simulink model "MPC"  (R2024b)
settings: Solver=ode4  StartTime=0.0  StopTime=tsim  FixedStep=baseRate  RelTol=1e-6  AbsTol=1e-6
values from neighbouring files (symbols this model uses):
  C = [cos(theta), -sin(theta) ... (first row only)    [Run_Initializer.m]    (also in plotBatch.m = quat2Rotm(q','scalarFirst'))
  camera_FOV = 40*d2r    (= 0.698131700798)    [Run_Initializer.m]
  camera_offset = [0.145, 0.087]'    [Run_Initializer.m]
  docking_face = [0 1]'    [Run_Initializer.m]
  docking_offset = [0 0 0]'    [Run_Initializer.m]
  eta = 0.7    [Run_Initializer.m]
  F_t = [kron(eye(N_h),  [zeros(2,3), eye(2), zeros(2,4)]) ... (first row only)    [Run_Initializer.m]
  f_t = [kron(ones(N_h, 1), [xLength yLength]' - edge_buffer) ... (first row only)    [Run_Initializer.m]
  F_u = [kron(eye(N_h),  [eye(3), zeros(3,6)]) ... (first row only)    [Run_Initializer.m]
  f_u = kron(ones(2*N_h, 1), u_max')    [Run_Initializer.m]
  F_v = [kron(eye(N_h),  [zeros(1,5), 1, zeros(1,3)]) ... (first row only)    [Run_Initializer.m]
  gamma = 0.95    [Run_Initializer.m]
  Gamma1_el = 0.12    [Run_Initializer.m]
  Gamma1_sh = 0.005    [Run_Initializer.m]
  Gamma1_wr = 0.025    [Run_Initializer.m]
  Gamma2_el = 5    [Run_Initializer.m]
  Gamma2_sh = 5    [Run_Initializer.m]
  Gamma2_wr = 5    [Run_Initializer.m]
  Gamma3_el = 10    [Run_Initializer.m]
  Gamma3_sh = 40    [Run_Initializer.m]
  Gamma3_wr = 40    [Run_Initializer.m]
  Gamma4_el = 0.039    [Run_Initializer.m]
  Gamma4_sh = 0.015    [Run_Initializer.m]
  Gamma4_wr = 0.029    [Run_Initializer.m]
  Gamma5_el = 800    [Run_Initializer.m]
  Gamma5_sh = 800    [Run_Initializer.m]
  Gamma5_wr = 800    [Run_Initializer.m]
  Gamma6_el = 0.000001    (= 1e-06)    [Run_Initializer.m]
  Gamma6_sh = 0.005    [Run_Initializer.m]
  Gamma6_wr = 0.02    [Run_Initializer.m]
  H = kron(eye(N_h), [R, zeros(3,6); zeros(6,3), Q])    [Run_Initializer.m]
  IBLACK = 0.1996    [unpackData.m]
  IRED = 0.1982    [unpackData.m]
  J = sum(wp*posErr + wt*angErr)    [find_transformation.m]
  Kd_elarm = 0.8    [Run_Initializer.m]
  Kd_sharm = 1.0    (= 1)    [Run_Initializer.m]
  Kd_wrarm = 0.6    [Run_Initializer.m]
  Kp_elarm = 1.2    [Run_Initializer.m]
  Kp_sharm = 1.5    [Run_Initializer.m]
  Kp_wrarm = 1.0    (= 1)    [Run_Initializer.m]
  m = m + 5    (= 4)    [unpackData.m]
  M = diag([1/m; 1/m; 1/I])    [unpackData.m]
  maxd = [d1 ... (first row only)    [Run_Initializer.m]
  mBLACK = 11.3620    (= 11.362)    [unpackData.m]
  mRED = 11.2970    (= 11.297)    [unpackData.m]
  N = size(rel,1)    [plotBatch.m]    (also in unpackData.m = 0)
  p = [0 obj.pos(k,:)]    [SparseState6DOF.m]
  PDQ = blkdiag(20*eye(3),eye(3), 20*eye(3),eye(3))    [Run_Initializer.m]
  PQ = blkdiag(20*eye(6),eye(6))    [Run_Initializer.m]
  PR = blkdiag(20*eye(3), eye(6), 0.0001*eye(3))    [Run_Initializer.m]
  PWMFreq = 5    [Run_Initializer.m]
  Q = diag([100 100 100 300 300 300])    [Run_Initializer.m]    (also in unpackData.m = blkdiag(0.0001*eye(2), 0.00001))
  R = diag([200 200 200])    [Run_Initializer.m]    (also in plotBatch.m = C3(yaw); unpackData.m = diag([6;6;6]))
  r_hold_obs = 1.1*sqrt(2)*0.3.*[1 1]    [Run_Initializer.m]
  r_hold_tar_min = [0.8; (0.3+0.05)]    [Run_Initializer.m]
  rho = 0.98    [Run_Initializer.m]
  T_d = 2    [Run_Initializer.m]
  T_max = 0.15    [Run_Initializer.m]
  Tz_lim_elarm = .1    (= 0.1)    [Run_Initializer.m]
  Tz_lim_sharm = .1    (= 0.1)    [Run_Initializer.m]
  Tz_lim_wrarm = .1    (= 0.1)    [Run_Initializer.m]
  use_LOS_constr = 1    [Run_Initializer.m]
  use_table_constr = 1    [Run_Initializer.m]
  x_BLACK_0 = [(1/3)*xLength (1/3)*yLength-0.2 280*d2r 0.01 0.005 1.88*d2r]'    [Run_Initializer.m]
  x_BLUE_0 = [0 0 0 0 0 0]'    [Run_Initializer.m]
  zeta = 10*d2r    (= 0.174532925199)    [Run_Initializer.m]
undefined symbols (not defined in the file or in its folder): a1, a2, a3, alpha, alpha_m, alpha_t, alphas, alphas_t, alphat, Am, b, b0, b1, b2, b3, baseRate, Bm, c, c1, c1t, c2, c2t, Cm, d, dataRate, DiscIntNeverNeededParam, Dm, drop_states_ARM, drop_states_BLACK, drop_states_BLUE, drop_states_RED, epsilon, epsilont, F_black_X_nominal, F_black_Y_nominal, F_blue_X_nominal, F_blue_Y_nominal, F_max, F_red_X_nominal, F_red_Y_nominal, F_thrusters_BLACK, F_thrusters_BLUE, F_thrusters_RED, gamma_I, gamma_I_t, gamma_P, gamma_P_t, home_states_BLACK, home_states_BLUE, home_states_RED, IBLUE, IDIST, IEE, init_states_BLACK, init_states_BLUE, init_states_RED, IPROX, k, K, k1 ... (+62)
libraries: simulink x33, nvidiaSharedBlocks x13, slpidlib x6, MainLibrary x5, dspsigops x3, dspinverses x3, nvidiaIMUSensorslib x1
(part 11 of 12)

== matlab function MPC/4 - Control/Default PD Control (RED)/Sat/MATLAB Function5 ==
  data: q2 input; u input; saturation output; e parameter; T_max parameter; d parameter; J parameter
function saturation = fcn(q2,u,e, T_max, d, J)

if u >= e
    u = e;
elseif u <= -1*e
    u = -1*e;
else
    u = u;
end

u = d*q2*J + u;

if u >= T_max
    u = T_max;
elseif u <= -1*T_max
    u = -1*T_max;
else
    u = u;
end

saturation = u;

== matlab function MPC/4 - Control/Default PD Control (RED)/USC/MATLAB Function ==
  data: q1 input; k_dot output; q2 input; c1 parameter; c2 parameter
function k_dot = fcn(q1,q2,c1, c2)
k_dot = (q1*c1 + q2*c2)^2;
end

== matlab function MPC/4 - Control/Default PD Control (RED)/USC/MATLAB Function1 ==
  data: k input; q2 input; q1 input; u output; c1 parameter; c2 parameter
function u = fcn(k,q2,q1,c1, c2)
u = log(k)*(q1*c1 + q2*c2)*cos(sqrt(log(k)));
end

== matlab function MPC/4 - Control/Default PD Control (RED)/USC/MATLAB Function2 ==
  data: q1 input; k_dot output; q2 input; c1 parameter; c2 parameter
function k_dot = fcn(q1,q2,c1, c2)
k_dot = (q1*c1 + q2*c2)^2;
end

== matlab function MPC/4 - Control/Default PD Control (RED)/USC/MATLAB Function3 ==
  data: k input; q2 input; q1 input; u output; c1 parameter; c2 parameter
function u = fcn(k,q2,q1,c1, c2)
u = log(k)*(q1*c1 + q2*c2)*cos(sqrt(log(k)));
end

== matlab function MPC/4 - Control/Default PD Control (RED)/USC/MATLAB Function4 ==
  data: q1 input; k_dot output; q2 input; c1t parameter; c2t parameter
function k_dot = fcn(q1,q2,c1t, c2t)
k_dot = (q1*c1t + q2*c2t)^2;
end

== matlab function MPC/4 - Control/Default PD Control (RED)/USC/MATLAB Function5 ==
  data: k input; q2 input; q1 input; u output; c1t parameter; c2t parameter
function u = fcn(k,q2,q1,c1t, c2t)
u = log(k)*(q1*c1t + q2*c2t)*cos(sqrt(log(k)));
end

== matlab function MPC/4 - Control/Default PD Control (RED)/SAC/SAC_CTL/Position/Storage/MATLAB Function4 ==
  data: u input; y1 output; y2 output
function [y1,y2] = fcn(u)

y1 = u(1,:);
y2 = u(2,:);
end

== matlab function MPC/3 - Navigation/Subsystem/Filter Error/MATLAB Function2 ==
  data: true input; y output; est input
function y = fcn(true, est)
true(1:4) = normalizeQuat(true(1:4),'scalarFirst');
q = quatInv(true(1:4),'scalarFirst');
q = quatMultiply(q,est(1:4),'scalarFirst');
q = smallQuat(q,'scalarFirst');
mrp = quat2mrp(q,1,1,'scalarFirst');

temp = true(5:end) - est(5:end);

y = [mrp(3); temp(1:2); temp(6); temp(7:8)];

== matlab function MPC/3 - Navigation/Subsystem/Filter Error/MATLAB Function3 ==
  data: u input; y output; data input
function y = fcn(u, data)
y = quatMultiply(data,u,'scalarFirst');
y = smallQuat(y,'scalarFirst');

== matlab function MPC/3 - Navigation/Subsystem/Filter Error/MATLAB Function4 ==
  data: true input; y output; est input
function y = fcn(true, est)
true(1:4) = normalizeQuat(true(1:4),'scalarFirst');
q = quatInv(true(1:4),'scalarFirst');
q = quatMultiply(q,est(1:4),'scalarFirst');
q = smallQuat(q,'scalarFirst');
mrp = quat2mrp(q,1,1,'scalarFirst');

temp = true(5:end) - est(5:end);

y = [mrp(3); temp(1:2); temp(6); temp(7:8)];

== matlab function MPC/3 - Navigation/Subsystem/Filter Error/MATLAB Function5 ==
  data: q input; y output; v input; x input
function y = fcn(q, v, x)
t = 0.75;
t = 0;
a = [0;0;1;t*pi/180];
d = axang2Quat(a,'scalarFirst');
d = normalizeQuat(d,'scalarFirst');
q = normalizeQuat(q,'scalarFirst');
q = quatMultiply(d,q,'scalarFirst');
v = quatRotate(q,v,'scalarFirst');
y = v + x;

== matlab function MPC/3 - Navigation/Subsystem/Filter Error/MATLAB Function6 ==
  data: true input; y output; est input
function y = fcn(true, est)
true(1:4) = normalizeQuat(true(1:4),'scalarFirst');
q = quatInv(true(1:4),'scalarFirst');
q = quatMultiply(q,est(1:4),'scalarFirst');
q = smallQuat(q,'scalarFirst');
mrp = quat2mrp(q,1,1,'scalarFirst');

temp = true(5:end) - est(5:end);

y = [mrp(3); temp(1:2); temp(6); temp(7:8)];

== matlab function MPC/3 - Navigation/Subsystem/Filter Error/MATLAB Function7 ==
  data: true input; y output; est input
function y = fcn(true, est)
true(1:4) = normalizeQuat(true(1:4),'scalarFirst');
q = quatInv(true(1:4),'scalarFirst');
q = quatMultiply(q,est(1:4),'scalarFirst');
q = smallQuat(q,'scalarFirst');
mrp = quat2mrp(q,1,1,'scalarFirst');

temp = true(5:end) - est(5:end);
y = [mrp(3); temp(1); temp(2);];

== matlab function MPC/3 - Navigation/Subsystem/Filter Error/MATLAB Function8 ==
  data: true input; y output; est input
function y = fcn(true, est)
true(1:4) = normalizeQuat(true(1:4),'scalarFirst');
q = quatInv(true(1:4),'scalarFirst');
q = quatMultiply(q,est(1:4),'scalarFirst');
q = smallQuat(q,'scalarFirst');
mrp = quat2mrp(q,1,1,'scalarFirst');

temp = true(5:end) - est(5:end);

y = [mrp(3); temp(1:2); temp(6); temp(7:8)];

== matlab function MPC/3 - Navigation/Subsystem/Representations/MATLAB Function ==
  data: u input; dq output; q output; R output; x output; v output; w output; yaw output
function [dq,q,R,x,v,w,yaw] = fcn(u)
    v = u(7:9);
    w = u(10:12);
    x = u(1:3);
    R = C3(u(6));
    yaw = u(6);
    T = [R, x; zeros(1,3), 1];
    T = htformInverse(T);
    q = rotm2Quat(R,'scalarFirst');
    q = smallQuat(q,'scalarFirst');
    dq = htform2Dq(T,'scalarFirst');
end

== matlab function MPC/3 - Navigation/Subsystem/Representations1/MATLAB Function ==
  data: u input; dq output; q output; R output; x output; v output; w output; yaw output
function [dq,q,R,x,v,w,yaw] = fcn(u)
    v = u(7:9);
    w = u(10:12);
    x = u(1:3);
    R = C3(u(6));
    yaw = u(6);
    T = [R, x; zeros(1,3), 1];
    q = rotm2Quat(R,'scalarFirst');
    q = smallQuat(q,'scalarFirst');
    dq = htform2Dq(T,'scalarFirst');
end

== matlab function MPC/2 - Guidance/Default APF PPL (RED)/MATLAB Function ==
  data: desiredPosition input; currentPosition output; currentPosition input; obstacles input; attractiveGain input; repulsiveGain input; influenceRange input; angularGain input; baseRate parameter
function currentPosition = APFPathPlanner(desiredPosition, currentPosition, obstacles, attractiveGain, repulsiveGain, influenceRange, angularGain, baseRate)
    % APFPathPlanner for real-time path planning in Simulink
    % Controls X, Y, and Attitude (Theta)
    % currentPosition: [x, y, theta]
    % desiredPosition: [x, y, theta]
    % obstacles: Nx2 matrix of obstacle positions [x, y]
    % attractiveGain: Scalar for attractive force
    % repulsiveGain: Scalar for repulsive force
    % influenceRange: Scalar, range for obstacle influence
    % angularGain: Scalar for angular adjustment


    % Position control for X and Y
    attractiveForce = attractiveGain * (desiredPosition(1:2) - currentPosition(1:2));
    repulsiveForce = zeros(1, 2);

    % % Repulsive force from obstacles
    for i = 1:size(obstacles, 1)
        obstaclePos = obstacles(i, :);
        distanceToObstacle = norm(currentPosition(1:2) - obstaclePos);

        if distanceToObstacle < influenceRange
            directionFromObstacle = (currentPosition(1:2) - obstaclePos) / distanceToObstacle;
            magnitude = repulsiveGain * (1 / distanceToObstacle - 1 / influenceRange) * (1 / distanceToObstacle^2);
            repulsiveForce = repulsiveForce + magnitude * directionFromObstacle;
        end
    end

    % Combine attractive and repulsive forces
    totalForce = attractiveForce + repulsiveForce;

    % Update X and Y position
    deltaT = baseRate;
    newPosition = currentPosition(1:2) + deltaT * totalForce;

    % Attitude control for Theta
    angularDifference = atan2(sin(desiredPosition(3) - currentPosition(3)), cos(desiredPosition(3) - currentPosition(3)));
    newTheta = currentPosition(3) + angularGain * angularDifference * deltaT;

    % Normalize newTheta to be within -pi to pi
    newTheta = atan2(sin(newTheta), cos(newTheta));

    % Update currentPosition with new position and attitude
    currentPosition = [newPosition, newTheta];

end

== matlab function MPC/3 - Navigation/Subsystem/MATLAB Function ==
  data: u input; states output
function states = fcn(u)

x = u(1);
y = u(2);
z = 0;
roll = 0;
pitch = 0;
yaw = u(3);
dx = u(4);
dy = u(5);
dz = 0;
droll = 0;
dpitch = 0;
dyaw = u(6);

states = [x; y; z; ...
          roll; pitch; yaw; ...
          dx; dy; dz; ...
          droll; dpitch; dyaw];

== matlab function MPC/3 - Navigation/Subsystem/MATLAB Function1 ==
  data: u input; states output
function states = fcn(u)

x = u(1);
y = u(2);
z = 0;
roll = 0;
pitch = 0;
yaw = u(3);
dx = u(4);
dy = u(5);
dz = 0;
droll = 0;
dpitch = 0;
dyaw = u(6);

states = [x; y; z; ...
          roll; pitch; yaw; ...
          dx; dy; dz; ...
          droll; dpitch; dyaw];

== matlab function MPC/PhaseSpace Camera Code/Use Hardware to Obtain States/Store RED Data/Subsystem1/Enabled Subsystem/MATLAB Function ==
  data: y input; dy output; dt input; tau input; dy_prev input; ema_prev input; ema output
function [dy, ema] = realtime_derivative_ema(y, dt, tau, dy_prev, ema_prev)
    % Inputs:
    % y: Current measurement
    % dt: Time step
    % alpha: Smoothing factor (e.g., 0.1)

    alpha = 1 - exp(-dt / tau);
        
    % Update EMA
    ema = alpha.*y + (1 - alpha).*ema_prev;
    
    % Compute derivative
    dy = (ema - ema_prev)./dt;
    
end

== matlab function MPC/Simulate Plant Dynamics/BLACK Dynamics/Calculated & Store Measured States/Subsystem2/Enabled Subsystem/MATLAB Function ==
  data: y input; dy output; dt input; tau input; dy_prev input; ema_prev input; ema output
function [dy, ema] = realtime_derivative_ema(y, dt, tau, dy_prev, ema_prev)
    % Inputs:
    % y: Current measurement
    % dt: Time step
    % alpha: Smoothing factor (e.g., 0.1)

    alpha = 1 - exp(-dt / tau);
        
    % Update EMA
    ema = alpha.*y + (1 - alpha).*ema_prev;
    
    % Compute derivative
    dy = (ema - ema_prev)./dt;
    
end

== matlab function MPC/Simulate Plant Dynamics/RED and ARM Dynamics/RED + ARM/Coriolis Function1 ==
  data: a1 parameter; a2 parameter; a3 parameter; b0 parameter; b1 parameter; b2 parameter; mPROX parameter; mDIST parameter; mEE parameter; Phi parameter; CoriolisS output; x input
function CoriolisS = CoriolisFunc3LINK(a1,a2,a3,b0,b1,b2,mPROX,mDIST,mEE,Phi,x)
%CORIOLISFUNC3LINK
%    CORIOLISS = CORIOLISFUNC3LINK(A1,A2,A3,B0,B1,B2,mPROX,mDIST,mEE,PHI,Q0,Q1,Q2,Q3,Q0_DOT,Q1_DOT,Q2_DOT,Q3_DOT)

%    This function was generated by the Symbolic Math Toolbox version 8.0.
%    05-Nov-2017 11:48:44

q0 = x(3);
q1 = x(4);
q2 = x(5);
q3 = x(6);

q0_dot = x(9);
q1_dot = x(10);
q2_dot = x(11);
q3_dot = x(12);

t2 = a1+b1;
t3 = a1.*mPROX;
t4 = mDIST.*t2;
t5 = mEE.*t2;
t6 = t3+t4+t5;
t7 = a2.*mDIST;
t8 = a2+b2;
t9 = mEE.*t8;
t10 = t7+t9;
t11 = pi.*(1.0./2.0);
t12 = q0_dot.*t6;
t13 = q1_dot.*t6;
t14 = q0+q1+t11;
t15 = cos(t14);
t16 = t12+t13;
t17 = q0_dot.*t10;
t18 = q1_dot.*t10;
t19 = q2_dot.*t10;
t20 = q0+q1+q2+t11;
t21 = cos(t20);
t22 = t17+t18+t19;
t23 = a3.*mEE.*q0_dot;
t24 = a3.*mEE.*q1_dot;
t25 = a3.*mEE.*q2_dot;
t26 = a3.*mEE.*q3_dot;
t27 = q0+q1+q2+q3+t11;
t28 = cos(t27);
t29 = t23+t24+t25+t26;
t30 = b0.*mPROX;
t31 = b0.*mDIST;
t32 = b0.*mEE;
t33 = t30+t31+t32;
t34 = (pi/2-Phi)+q0;
t35 = sin(t14);
t36 = sin(t20);
t37 = sin(t27);
t38 = q0_dot+q1_dot+q2_dot+q3_dot;
t39 = q0+q1+q2+q3;
t40 = a1.*b0.*mPROX.*q1_dot;
t41 = a1.*b0.*mDIST.*q1_dot;
t42 = a1.*b0.*mEE.*q1_dot;
t43 = b0.*b1.*mDIST.*q1_dot;
t44 = b0.*b1.*mEE.*q1_dot;
t45 = (pi/2-Phi)-q1;
t46 = cos(t45);
t47 = a2.*b0.*mDIST.*q1_dot;
t48 = a2.*b0.*mDIST.*q2_dot;
t49 = a2.*b0.*mEE.*q1_dot;
t50 = a2.*b0.*mEE.*q2_dot;
t51 = b0.*b2.*mEE.*q1_dot;
t52 = b0.*b2.*mEE.*q2_dot;
t53 = -(pi/2-Phi)+q1+q2;
t54 = cos(t53);
t55 = a3.*b0.*mEE.*q1_dot;
t56 = a3.*b0.*mEE.*q2_dot;
t57 = a3.*b0.*mEE.*q3_dot;
t58 = -(pi/2-Phi)+q1+q2+q3;
t59 = cos(t58);
t60 = a2.*b1.*mDIST.*q2_dot;
t61 = a1.*b2.*mEE.*q2_dot;
t62 = a2.*b1.*mEE.*q2_dot;
t63 = b1.*b2.*mEE.*q2_dot;
t64 = a1.*a2.*mDIST.*q2_dot;
t65 = a1.*a2.*mEE.*q2_dot;
t66 = sin(q2);
t67 = t60+t61+t62+t63+t64+t65;
t68 = a3.*b2.*mEE.*q3_dot;
t69 = a2.*a3.*mEE.*q3_dot;
t70 = sin(q3);
t71 = t68+t69;
t72 = a3.*b1.*mEE.*q2_dot;
t73 = a3.*b1.*mEE.*q3_dot;
t74 = a1.*a3.*mEE.*q2_dot;
t75 = a1.*a3.*mEE.*q3_dot;
t76 = q2+q3;
t77 = sin(t76);
t78 = t72+t73+t74+t75;
t79 = a2.*b0.*mDIST.*q0_dot;
t80 = a2.*b0.*mEE.*q0_dot;
t81 = b0.*b2.*mEE.*q0_dot;
t82 = t47+t48+t49+t50+t51+t52+t79+t80+t81;
t83 = a3.*b0.*mEE.*q0_dot;
t84 = t55+t56+t57+t83;
t85 = a1.*b0.*mPROX.*q0_dot;
t86 = a1.*b0.*mDIST.*q0_dot;
t87 = a1.*b0.*mEE.*q0_dot;
t88 = b0.*b1.*mDIST.*q0_dot;
t89 = b0.*b1.*mEE.*q0_dot;
t90 = a2.*b1.*mDIST.*q0_dot;
t91 = a1.*b2.*mEE.*q0_dot;
t92 = a2.*b1.*mDIST.*q1_dot;
t93 = a2.*b1.*mEE.*q0_dot;
t94 = a1.*b2.*mEE.*q1_dot;
t95 = a2.*b1.*mEE.*q1_dot;
t96 = b1.*b2.*mEE.*q0_dot;
t97 = b1.*b2.*mEE.*q1_dot;
t98 = a1.*a2.*mDIST.*q0_dot;
t99 = a1.*a2.*mDIST.*q1_dot;
t100 = a1.*a2.*mEE.*q0_dot;
t101 = a1.*a2.*mEE.*q1_dot;
t102 = t60+t61+t62+t63+t64+t65+t90+t91+t92+t93+t94+t95+t96+t97+t98+t99+t100+t101;
t103 = a3.*b1.*mEE.*q0_dot;
t104 = a3.*b1.*mEE.*q1_dot;
t105 = a1.*a3.*mEE.*q0_dot;
t106 = a1.*a3.*mEE.*q1_dot;
t107 = t72+t73+t74+t75+t103+t104+t105+t106;
t108 = t79+t80+t81;
t109 = t54.*t108;
t110 = t59.*t83;
t111 = t90+t91+t92+t93+t94+t95+t96+t97+t98+t99+t100+t101;
t112 = t66.*t111;
t113 = t103+t104+t105+t106;
t114 = t77.*t113;
t115 = a2.*q0_dot;
t116 = a2.*q1_dot;
t117 = a2.*q2_dot;
t118 = b2.*q0_dot;
t119 = b2.*q1_dot;
t120 = b2.*q2_dot;
t121 = t115+t116+t117+t118+t119+t120;
t122 = a3.*mEE.*t70.*t121;
t123 = a1.*q0_dot;
t124 = a1.*q1_dot;
t125 = b1.*q0_dot;
t126 = b1.*q1_dot;
t127 = t123+t124+t125+t126;
t128 = a3.*mEE.*t77.*t127;
CoriolisS = reshape([0.0,0.0,0.0,0.0,0.0,0.0,0.0,0.0,0.0,0.0,0.0,0.0,-t15.*t16-t21.*t22-t28.*t29-q0_dot.*t33.*cos(t34),-t16.*t35-t22.*t36-t29.*t37-q0_dot.*t33.*sin(t34),-t66.*t67-t70.*t71-t77.*t78-t46.*(t40+t41+t42+t43+t44)-t59.*(t55+t56+t57)-t54.*(t47+t48+t49+t50+t51+t52),t109+t110-t66.*t67-t70.*t71-t77.*t78+t46.*(t85+t86+t87+t88+t89),t109+t110+t112+t114-t70.*t71,t110+t122+t128,-t15.*t16-t21.*t22-t28.*t29,-t16.*t35-t22.*t36-t29.*t37,-t66.*t67-t54.*t82-t70.*t71-t59.*t84-t77.*t78-t46.*(t40+t41+t42+t43+t44+t85+t86+t87+t88+t89),-t66.*t67-t70.*t71-t77.*t78,t112+t114-t70.*t71,t122+t128,-t21.*t22-t28.*t29,-t22.*t36-t29.*t37,-t54.*t82-t70.*t71-t59.*t84-t66.*t102-t77.*t107,-t70.*t71-t66.*t102-t77.*t107,-a3.*mEE.*q3_dot.*t8.*t70,a3.*mEE.*t8.*t70.*(q0_dot+q1_dot+q2_dot),a3.*mEE.*t38.*sin(t39),-a3.*mEE.*t38.*cos(t39),-a3.*b0.*mEE.*t38.*t59-a3.*mEE.*t8.*t38.*t70-a3.*mEE.*t2.*t38.*t77,-a3.*mEE.*t8.*t38.*t70-a3.*mEE.*t2.*t38.*t77,-a3.*mEE.*t8.*t38.*t70,0.0],[6,6]);
end

== matlab function MPC/Simulate Plant Dynamics/BLACK Dynamics/Data @ Measurement Rate/Calculate True Time Step/MATLAB Function ==
  data: dt input; dt_out output; dataRate input
function dt_out = CheckforInvalidTime(dt, dataRate)

    if dt <= 0

        dt_out = dataRate;

    else

        dt_out = dt;

    end


end

== matlab function MPC/Simulate Plant Dynamics/RED and ARM Dynamics/RED + ARM/Inertia Function 1 ==
  data: mRED parameter; IRED parameter; Phi parameter; b0 parameter; a1 parameter; b1 parameter; a2 parameter; b2 parameter; a3 parameter; b3 parameter; mPROX parameter; mDIST parameter; mEE parameter; IPROX parameter; IDIST parameter; InertiaS output; x input; IEE parameter
function InertiaS = InertiaFunc3LINK(mRED, IRED, Phi, b0, a1, b1, a2, b2, a3, b3, mPROX, mDIST, mEE, IPROX, IDIST, x, IEE)

    q0 = x(3);
    q1 = x(4);
    q2 = x(5);
    q3 = x(6);
    
    t2 = a1+b1;
    t3 = a1.*mPROX;
    t4 = mDIST.*t2;
    t5 = mEE.*t2;
    t6 = q0+q1;
    t7 = cos(t6);
    t8 = t3+t4+t5;
    t9 = a2.*mDIST;
    t10 = a2+b2;
    t11 = mEE.*t10;
    t12 = q0+q1+q2;
    t13 = cos(t12);
    t14 = t9+t11;
    t15 = q0+q1+q2+q3;
    t16 = cos(t15);
    t17 = mRED+mPROX+mDIST+mEE;
    t18 = b0.*mPROX;
    t19 = b0.*mDIST;
    t20 = b0.*mEE;
    t21 = t18+t19+t20;
    t22 = (pi/2-Phi)+q0;
    t23 = sin(t6);
    t24 = sin(t12);
    t25 = sin(t15);
    t26 = a2.*mEE;
    t27 = b2.*mEE;
    t28 = t9+t26+t27;
    t29 = sin(t22);
    t86 = t7.*t8;
    t87 = t13.*t14;
    t88 = a3.*mEE.*t16;
    t30 = -t86-t87-t88-t21.*t29;
    t31 = cos(t22);
    t32 = t21.*t31;
    t89 = t8.*t23;
    t90 = t14.*t24;
    t91 = a3.*mEE.*t25;
    t33 = t32-t89-t90-t91;
    t34 = a1.^2;
    t35 = a2.^2;
    t36 = b0.^2;
    t37 = b1.^2;
    t38 = a1.*a2.*mDIST.*2.0;
    t39 = a1.*a2.*mEE.*2.0;
    t40 = a2.*b1.*mDIST.*2.0;
    t41 = a1.*b2.*mEE.*2.0;
    t42 = a2.*b1.*mEE.*2.0;
    t43 = b1.*b2.*mEE.*2.0;
    t44 = t38+t39+t40+t41+t42+t43;
    t45 = cos(q2);
    t46 = t44.*t45;
    t47 = a2.*a3.*mEE.*2.0;
    t48 = a3.*b2.*mEE.*2.0;
    t49 = t47+t48;
    t50 = cos(q3);
    t51 = t49.*t50;
    t52 = a1.*a3.*mEE.*2.0;
    t53 = a3.*b1.*mEE.*2.0;
    t54 = t52+t53;
    t55 = q2+q3;
    t56 = cos(t55);
    t57 = t54.*t56;
    t58 = (pi/2-Phi)-q1;
    t59 = sin(t58);
    t60 = -(pi/2-Phi)+q1+q2;
    t61 = sin(t60);
    t62 = -(pi/2-Phi)+q1+q2+q3;
    t63 = sin(t62);
    t64 = mPROX.*t34;
    t65 = mDIST.*t34;
    t66 = mEE.*t34;
    t67 = mDIST.*t35;
    t68 = mEE.*t35;
    t69 = a3.^2;
    t70 = mEE.*t69;
    t71 = mDIST.*t37;
    t72 = mEE.*t37;
    t73 = b2.^2;
    t74 = mEE.*t73;
    t75 = a1.*b1.*mDIST.*2.0;
    t76 = a1.*b1.*mEE.*2.0;
    t77 = a2.*b2.*mEE.*2.0;
    t78 = a2.*b0.*mDIST;
    t79 = a2.*b0.*mEE;
    t80 = b0.*b2.*mEE;
    t81 = t78+t79+t80;
    t82 = a1.*a3.*mEE;
    t83 = a3.*b1.*mEE;
    t84 = t82+t83;
    t85 = t56.*t84;
    t92 = a1.*b0.*mPROX;
    t93 = a1.*b0.*mDIST;
    t94 = a1.*b0.*mEE;
    t95 = b0.*b1.*mDIST;
    t96 = b0.*b1.*mEE;
    t97 = t92+t93+t94+t95+t96;
    t98 = t59.*t97;
    t112 = t61.*t81;
    t113 = a3.*b0.*mEE.*t63;
    t99 = IPROX+IDIST+IEE+t46+t51+t57+t64+t65+t66+t67+t68+t70+t71+t72+t74+t75+t76+t77+t98-t112-t113;
    t100 = a1.*a2.*mDIST;
    t101 = a1.*a2.*mEE;
    t102 = a2.*b1.*mDIST;
    t103 = a1.*b2.*mEE;
    t104 = a2.*b1.*mEE;
    t105 = b1.*b2.*mEE;
    t106 = t100+t101+t102+t103+t104+t105;
    t107 = t45.*t106;
    t108 = a2.*a3.*mEE;
    t109 = a3.*b2.*mEE;
    t110 = t108+t109;
    t111 = t50.*t110;
    t114 = IDIST+IEE+t51+t67+t68+t70+t74+t77+t85+t107;
    t115 = IEE+t70+t85+t111;
    t116 = IEE+t70+t111;
    InertiaS = reshape([t17,0.0,t30,-t86-t87-t88,-t88-t13.*t28,-t88,0.0,t17,t33,-t89-t90-t91,-t91-t24.*t28,-t91,t30,t33,IRED+IPROX+IDIST+IEE+t46+t51+t57+t64+t65+t66+t67+t68+t70+t71+t72+t74+t75+t76+t77+t59.*(a1.*b0.*mPROX.*2.0+a1.*b0.*mDIST.*2.0+a1.*b0.*mEE.*2.0+b0.*b1.*mDIST.*2.0+b0.*b1.*mEE.*2.0)+mPROX.*t36+mDIST.*t36+mEE.*t36-t61.*(a2.*b0.*mDIST.*2.0+a2.*b0.*mEE.*2.0+b0.*b2.*mEE.*2.0)-a3.*b0.*mEE.*t63.*2.0,t99,IDIST+IEE+t51+t67+t68+t70+t74+t77+t85+t107-t112-t113,IEE+t70+t85+t111-t113,-t7.*t8-t13.*t14-a3.*mEE.*t16,-t8.*t23-t14.*t24-a3.*mEE.*t25,t99,IPROX+IDIST+IEE+t46+t51+t57+t64+t65+t66+t67+t68+t70+t71+t72+t74+t75+t76+t77,t114,t115,-t13.*t28-a3.*mEE.*t16,-t24.*t28-a3.*mEE.*t25,IDIST+IEE+t51+t67+t68+t70+t74+t77+t85+t107-t61.*t81-a3.*b0.*mEE.*t63,t114,IDIST+IEE+t51+t67+t68+t70+t74+t77,t116,-a3.*mEE.*t16,-a3.*mEE.*t25,IEE+t70+t85+t111-a3.*b0.*mEE.*t63,t115,t116,IEE+t70],[6,6]);
end

== matlab function MPC/Simulate Plant Dynamics/BLUE Dynamics/Calculated & Store Measured States/Subsystem1/Enabled Subsystem/MATLAB Function ==
  data: y input; dy output; dt input; tau input; dy_prev input; ema_prev input; ema output
function [dy, ema] = realtime_derivative_ema(y, dt, tau, dy_prev, ema_prev)
    % Inputs:
    % y: Current measurement
    % dt: Time step
    % alpha: Smoothing factor (e.g., 0.1)

    alpha = 1 - exp(-dt / tau);
        
    % Update EMA
    ema = alpha.*y + (1 - alpha).*ema_prev;
    
    % Compute derivative
    dy = (ema - ema_prev)./dt;
    
end

== matlab function MPC/Simulate Plant Dynamics/BLACK Dynamics/Dynamics Model for BLACK/MATLAB Function ==
  data: control_inputs input; x_ddot output; mBLACK parameter; IBLACK parameter
function x_ddot = BLACK_dynamics(control_inputs, mBLACK, IBLACK)

%#codegen
% Fully define the size of x_ddot() for code generation:
x_ddot     = zeros(3,1);

% Extract the control inputs from the control_input vector:
Fx        = control_inputs(1);              % [N]
Fy        = control_inputs(2);              % [N]
Tz        = control_inputs(3);              % [N.m]

% Calculate the state acceleration vector:
x_ddot(1) = Fx/mBLACK;                      % [m/s^2]
x_ddot(2) = Fy/mBLACK;                      % [m/s^2]
x_ddot(3) = Tz/IBLACK;                      % [rad/s^2]

end

== matlab function MPC/Simulate Plant Dynamics/BLUE Dynamics/BLUE  Dynamics Model/MATLAB Function ==
  data: control_inputs input; x_ddot output; mBLUE parameter; IBLUE parameter
function x_ddot = BLUE_dynamics(control_inputs, mBLUE, IBLUE)%#codegen
% Fully define the size of x_ddot() for code generation:
x_ddot     = zeros(3,1);

% Extract the control inputs from the control_input vector:
Fx        = control_inputs(1);              % [N]
Fy        = control_inputs(2);              % [N]
Tz        = control_inputs(3);              % [N.m]

% Calculate the state acceleration vector:
x_ddot(1) = Fx/mBLUE;                      % [m/s^2]
x_ddot(2) = Fy/mBLUE;                      % [m/s^2]
x_ddot(3) = Tz/IBLUE;                      % [rad/s^2]

end

== matlab function MPC/Gyro.//Accel. Code/Log Gyro//Accel/Parse IMU Data ==
  data: WhoAmI input; RED_IMU_Ax output; IMU_Ax input; IMU_Ay input; IMU_Gz input; RED_IMU_Ay output; RED_IMU_Gz output; BLACK_IMU_Ax output; BLACK_IMU_Ay output; BLACK_IMU_Gz output; BLUE_IMU_Ax output; BLUE_IMU_Ay output; BLUE_IMU_Gz output
function [RED_IMU_Ax, RED_IMU_Ay, RED_IMU_Gz, BLACK_IMU_Ax, BLACK_IMU_Ay, BLACK_IMU_Gz, BLUE_IMU_Ax, BLUE_IMU_Ay, BLUE_IMU_Gz] = ParseIMUData(WhoAmI, IMU_Ax, IMU_Ay, IMU_Gz)

    if WhoAmI == 1 % This is RED

        RED_IMU_Ax = IMU_Ax;
        RED_IMU_Ay = IMU_Ay;
        RED_IMU_Gz = IMU_Gz;
        BLACK_IMU_Ax = 0;
        BLACK_IMU_Ay = 0;
        BLACK_IMU_Gz = 0;
        BLUE_IMU_Ax = 0;
        BLUE_IMU_Ay = 0;
        BLUE_IMU_Gz = 0;

    elseif WhoAmI == 2 % This is BLACK

        RED_IMU_Ax = 0;
        RED_IMU_Ay = 0;
        RED_IMU_Gz = 0;
        BLACK_IMU_Ax = IMU_Ax;
        BLACK_IMU_Ay = IMU_Ay;
        BLACK_IMU_Gz = IMU_Gz;
        BLUE_IMU_Ax = 0;
        BLUE_IMU_Ay = 0;
        BLUE_IMU_Gz = 0;

    elseif WhoAmI == 3 % This is BLUE

        RED_IMU_Ax = 0;
        RED_IMU_Ay = 0;
        RED_IMU_Gz = 0;
        BLACK_IMU_Ax = 0;
        BLACK_IMU_Ay = 0;
        BLACK_IMU_Gz = 0;
        BLUE_IMU_Ax = IMU_Ax;
        BLUE_IMU_Ay = IMU_Ay;
        BLUE_IMU_Gz = IMU_Gz;

    else 

        RED_IMU_Ax = 0;
        RED_IMU_Ay = 0;
        RED_IMU_Gz = 0;
        BLACK_IMU_Ax = 0;
        BLACK_IMU_Ay = 0;
        BLACK_IMU_Gz = 0;
        BLUE_IMU_Ax = 0;
        BLUE_IMU_Ay = 0;
        BLUE_IMU_Gz = 0;       

    end

end

== matlab function MPC/Simulate Plant Dynamics/BLUE Dynamics/Calculated & Store Measured States/Subsystem2/Enabled Subsystem/MATLAB Function ==
  data: y input; dy output; dt input; tau input; dy_prev input; ema_prev input; ema output
function [dy, ema] = realtime_derivative_ema(y, dt, tau, dy_prev, ema_prev)
    % Inputs:
    % y: Current measurement
    % dt: Time step
    % alpha: Smoothing factor (e.g., 0.1)

    alpha = 1 - exp(-dt / tau);
        
    % Update EMA
    ema = alpha.*y + (1 - alpha).*ema_prev;
    
    % Compute derivative
    dy = (ema - ema_prev)./dt;
    
end

== matlab function MPC/Simulate Plant Dynamics/BLUE Dynamics/Data @ Measurement Rate/Calculate True Time Step/MATLAB Function ==
  data: dt input; dt_out output; dataRate input
function dt_out = CheckforInvalidTime(dt, dataRate)

    if dt <= 0

        dt_out = dataRate;

    else

        dt_out = dt;

    end


end

== matlab function MPC/Model Predictive Control/Model Predictive Control/Dynamics Constraint ==
  data: x_RED input; b output; A_d parameter
function b = fcn(x_RED, A_d)

% Define horizon length
N_h = 15;

% Compute b vector
b = [A_d*x_RED; zeros(6*(N_h-1),1)];

end

== matlab function MPC/PhaseSpace Camera Code/Use Hardware to Obtain States/Store RED Data/Subsystem2/Enabled Subsystem/MATLAB Function ==
  data: y input; dy output; dt input; tau input; dy_prev input; ema_prev input; ema output
function [dy, ema] = realtime_derivative_ema(y, dt, tau, dy_prev, ema_prev)
    % Inputs:
    % y: Current measurement
    % dt: Time step
    % alpha: Smoothing factor (e.g., 0.1)

    alpha = 1 - exp(-dt / tau);
        
    % Update EMA
    ema = alpha.*y + (1 - alpha).*ema_prev;
    
    % Compute derivative
    dy = (ema - ema_prev)./dt;
    
end

== matlab function MPC/PhaseSpace Camera Code/Use Hardware to Obtain States/Store BLACK Data/Calculate True Time Step/MATLAB Function ==
  data: dt input; dt_out output; dataRate input
function dt_out = CheckforInvalidTime(dt, dataRate)

    if dt <= 0

        dt_out = dataRate;

    else

        dt_out = dt;

    end


end

== matlab function MPC/PhaseSpace Camera Code/Use Hardware to Obtain States/Store RED Data/Calculate True Time Step/MATLAB Function ==
  data: dt input; dt_out output; dataRate input
function dt_out = CheckforInvalidTime(dt, dataRate)

    if dt <= 0

        dt_out = dataRate;

    else

        dt_out = dt;

    end


end

== matlab function MPC/PhaseSpace Camera Code/Use Hardware to Obtain States/Store BLACK Data/Subsystem1/Enabled Subsystem/MATLAB Function ==
  data: y input; dy output; dt input; tau input; dy_prev input; ema_prev input; ema output
function [dy, ema] = realtime_derivative_ema(y, dt, tau, dy_prev, ema_prev)
    % Inputs:
    % y: Current measurement
    % dt: Time step
    % alpha: Smoothing factor (e.g., 0.1)

    alpha = 1 - exp(-dt / tau);
        
    % Update EMA
    ema = alpha.*y + (1 - alpha).*ema_prev;
    
    % Compute derivative
    dy = (ema - ema_prev)./dt;
    
end

== matlab function MPC/PhaseSpace Camera Code/Use Hardware to Obtain States/Store BLACK Data/Subsystem2/Enabled Subsystem/MATLAB Function ==
  data: y input; dy output; dt input; tau input; dy_prev input; ema_prev input; ema output
function [dy, ema] = realtime_derivative_ema(y, dt, tau, dy_prev, ema_prev)
    % Inputs:
    % y: Current measurement
    % dt: Time step
    % alpha: Smoothing factor (e.g., 0.1)

    alpha = 1 - exp(-dt / tau);
        
    % Update EMA
    ema = alpha.*y + (1 - alpha).*ema_prev;
    
    % Compute derivative
    dy = (ema - ema_prev)./dt;
    
end

== matlab function MPC/PhaseSpace Camera Code/Use Hardware to Obtain States/Store BLUE Data/Calculate True Time Step/MATLAB Function ==
  data: dt input; dt_out output; dataRate input
function dt_out = CheckforInvalidTime(dt, dataRate)

    if dt <= 0

        dt_out = dataRate;

    else

        dt_out = dt;

    end


end

== matlab function MPC/PhaseSpace Camera Code/Use Hardware to Obtain States/Store BLUE Data/Subsystem1/Enabled Subsystem/MATLAB Function ==
  data: y input; dy output; dt input; tau input; dy_prev input; ema_prev input; ema output
function [dy, ema] = realtime_derivative_ema(y, dt, tau, dy_prev, ema_prev)
    % Inputs:
    % y: Current measurement
    % dt: Time step
    % alpha: Smoothing factor (e.g., 0.1)

    alpha = 1 - exp(-dt / tau);
        
    % Update EMA
    ema = alpha.*y + (1 - alpha).*ema_prev;
    
    % Compute derivative
    dy = (ema - ema_prev)./dt;
    
end

== matlab function MPC/PhaseSpace Camera Code/Use Hardware to Obtain States/Store BLUE Data/Subsystem2/Enabled Subsystem/MATLAB Function ==
  data: y input; dy output; dt input; tau input; dy_prev input; ema_prev input; ema output
function [dy, ema] = realtime_derivative_ema(y, dt, tau, dy_prev, ema_prev)
    % Inputs:
    % y: Current measurement
    % dt: Time step
    % alpha: Smoothing factor (e.g., 0.1)

    alpha = 1 - exp(-dt / tau);
        
    % Update EMA
    ema = alpha.*y + (1 - alpha).*ema_prev;
    
    % Compute derivative
    dy = (ema - ema_prev)./dt;
    
end

== matlab function MPC/Simulate Plant Dynamics/RED and ARM Dynamics/RED Only/Dynamics Model for RED/MATLAB Function ==
  data: control_inputs input; x_ddot output; mRED parameter; IRED parameter

    function x_ddot = RED_dynamics(control_inputs, mRED, IRED)

        %#codegen
        % Fully define the size of x_ddot() for code generation:
        x_ddot     = zeros(3,1);

        % Extract the servicer model parameters from the model_param vector defined
        % in initialize.m:

        % Extract the control inputs from the control_input vector:
        Fx        = control_inputs(1);              % [N]
        Fy        = control_inputs(2);              % [N]
        Tz        = control_inputs(3);              % [N.m]

        % Calculate the state acceleration vector:
        x_ddot(1) = Fx/mRED;                      % [m/s^2]
        x_ddot(2) = Fy/mRED;                      % [m/s^2]
        x_ddot(3) = Tz/IRED;                      % [rad/s^2]

    end

== matlab function MPC/Model Predictive Control/Model Predictive Control/Execute quadprog ==
  data: z_t input; P input; h input; H parameter; C parameter; b input; z output; z_0 input; u output; result output
% Solve the linear-quadratic optimization problem
function [z, u, result] = fcn(z_t, P, h, H, C, b, z_0)

% Compute equivalent cost function matrices
f = (-2.*z_t'*H)';
H = 2.*H;

% Configure solver options
options = optimoptions('quadprog', 'Algorithm', 'active-set', 'MaxIterations', 300);

% Run quadprog solver
tic
[z, ~, exitflag, output] = quadprog(H, f, P, h, C, b, [], [], z_0, options);
cputime = toc;

% Output solver results
result = [exitflag, output.iterations, cputime];

% Extract optimized control input for the current step
u = z(1:3);

== matlab function MPC/Model Predictive Control/Model Predictive Control/Propogate BLACK trajectory ==
  data: x_BLACK input; z_BLACK output; T_d parameter
% Compute expected trajectory of the target spacecraft
function z_BLACK = fcn(x_BLACK, T_d)

% Define horizon length
N_h = 15;

% Pre-allocate target trajectory variable
z_BLACK = zeros(9*N_h,1);

% Extract target velocities (assume constant velocity over the horizon)
v_BLACK = x_BLACK(4:6);

% Compute first entry with initial position
z_BLACK(4:9) = [x_BLACK(1:3) + v_BLACK.*T_d; v_BLACK];

% Iterate over the horizon
for j = 2:N_h
    row = 9*(j-1)+1;

    % Extract prior position
    pos_BLACK = z_BLACK(row-9+3:row-9+5);

    % Insert propogated position
    z_BLACK(row+3:row+9-1) = [pos_BLACK + v_BLACK.*T_d; v_BLACK];
end

end

== matlab function MPC/Model Predictive Control/Model Predictive Control/Propogate BLUE trajectory ==
  data: x_BLUE input; z_BLUE output; T_d parameter
% Compute expected trajectory of the target spacecraft
function z_BLUE = fcn(x_BLUE, T_d)

% Define horizon length
N_h = 15;

% Pre-allocate target trajectory variable
z_BLUE = zeros(9*N_h,1);

% Extract target velocities (assume constant velocity over the horizon)
v_BLUE = x_BLUE(4:6);

% Compute first entry with initial position
z_BLUE(4:9) = [x_BLUE(1:3) + v_BLUE.*T_d; v_BLUE];

% Iterate over the horizon
for j = 2:N_h
    row = 9*(j-1)+1;

    % Extract prior position
    pos_BLUE = z_BLUE(row-9+3:row-9+5);

    % Insert propogated position
    z_BLUE(row+3:row+9-1) = [pos_BLUE + v_BLUE.*T_d; v_BLUE];
end

end

== matlab function MPC/Simulate Plant Dynamics/RED and ARM Dynamics/RED + ARM/Data @ Measurement Rate/Calculate True Time Step/MATLAB Function ==
  data: dt input; dt_out output; dataRate input
function dt_out = CheckforInvalidTime(dt, dataRate)

    if dt <= 0

        dt_out = dataRate;

    else

        dt_out = dt;

    end


end

== matlab function MPC/Simulate Plant Dynamics/RED and ARM Dynamics/RED + ARM/Calculated & Store Measured States/Subsystem3/Enabled Subsystem/MATLAB Function ==
  data: y input; dy output; dt input; tau input; dy_prev input; ema_prev input; ema output
function [dy, ema] = realtime_derivative_ema(y, dt, tau, dy_prev, ema_prev)
    % Inputs:
    % y: Current measurement
    % dt: Time step
    % alpha: Smoothing factor (e.g., 0.1)

    alpha = 1 - exp(-dt / tau);
        
    % Update EMA
    ema = alpha.*y + (1 - alpha).*ema_prev;
    
    % Compute derivative
    dy = (ema - ema_prev)./dt;
    
end

== matlab function MPC/Model Predictive Control/Model Predictive Control/Update Holding Radius ==
  data: r_hold_tar input; x_RED input; x_BLACK input; r_hold_tar_min parameter; eta parameter; zeta parameter; gamma parameter; docking_face parameter; r_hold_tar output; docking_offset parameter; docking input; docking output
% Compute next holding radius
function [r_hold_tar, docking] = fcn(r_hold_tar, x_RED, x_BLACK, r_hold_tar_min, eta, zeta, gamma, docking_face, docking_offset, docking)

% Compute 2D z-axis rotation matrix representing the targets attitude
R = [cos(x_BLACK(3)) -sin(x_BLACK(3)); sin(x_BLACK(3)) cos(x_BLACK(3))];

% Compute the docking position in the global frame relative to the target
r_dock = R*(r_hold_tar(2).*docking_face + docking_offset(1:2));

% Compute the required attitude for docking
theta_star = x_BLACK(3) + docking_offset(3)-pi/2;

% Compute required chaser state for docking
x_t = [x_BLACK(1:2) + r_dock; theta_star];

% Compute positional and attitude errors
x_error = (x_RED(1:2) - x_t(1:2))'*(x_RED(1:2) - x_t(1:2));
theta_error = abs(atan2(sin(x_RED(3) - x_t(3)), cos(x_RED(3) - x_t(3))));

% Scale holding radius if tolerances are met
if x_error < eta^2 && theta_error < zeta
    r_hold_tar = gamma*r_hold_tar;
    docking = 1;
end

% Ensure holding radius does go below the defined minimum radius
r_hold_tar = max(r_hold_tar, r_hold_tar_min);

end

== matlab function MPC/Simulate Plant Dynamics/RED and ARM Dynamics/RED + ARM/Calculated & Store Measured States/Subsystem4/Enabled Subsystem/MATLAB Function ==
  data: y input; dy output; dt input; tau input; dy_prev input; ema_prev input; ema output
function [dy, ema] = realtime_derivative_ema(y, dt, tau, dy_prev, ema_prev)
    % Inputs:
    % y: Current measurement
    % dt: Time step
    % alpha: Smoothing factor (e.g., 0.1)

    alpha = 1 - exp(-dt / tau);
        
    % Update EMA
    ema = alpha.*y + (1 - alpha).*ema_prev;
    
    % Compute derivative
    dy = (ema - ema_prev)./dt;
    
end

== matlab function MPC/Simulate Plant Dynamics/RED and ARM Dynamics/RED + ARM/Calculated & Store Measured States/Subsystem5/Enabled Subsystem/MATLAB Function ==
  data: y input; dy output; dt input; tau input; dy_prev input; ema_prev input; ema output
function [dy, ema] = realtime_derivative_ema(y, dt, tau, dy_prev, ema_prev)
    % Inputs:
    % y: Current measurement
    % dt: Time step
    % alpha: Smoothing factor (e.g., 0.1)

    alpha = 1 - exp(-dt / tau);
        
    % Update EMA
    ema = alpha.*y + (1 - alpha).*ema_prev;
    
    % Compute derivative
    dy = (ema - ema_prev)./dt;
    
end

== matlab function MPC/Model Predictive Control/Model Predictive Control/Target Vision Constraint ==
  data: z_BLACK input; z_RED input; docking input; f_v output; docking_offset parameter; camera_FOV parameter; camera_offset parameter
 function f_v = fcn(z_BLACK, z_RED, docking, docking_offset, camera_FOV, camera_offset)

% Define horizon length
N_h = 15;

% Pre-allocate p vector
f_v = zeros(2*N_h,1);

% Iterate over the horizon
for j = 1:N_h
    pos = 9*(j-1)+1;

    R = [cos(z_RED(pos+5)), -sin(z_RED(pos+5)); 
         sin(z_RED(pos+5)),  cos(z_RED(pos+5))];

    % Compute relative position vector from camera to target
    r = z_BLACK(pos+3:pos+4) - z_RED(pos+3:pos+4) + R*camera_offset;

    % Compute desired pointing angle
    theta_star = rotateToFace(z_RED(pos+5), r) + docking_offset(3);

    if docking
        f_v(j) = theta_star + pi;
        f_v(j+N_h) = -1*(theta_star - pi);
    else
        f_v(j) = theta_star + (camera_FOV/2);
        f_v(j+N_h) = -1*(theta_star - (camera_FOV/2));
    end
end

end

%% Functions

function theta_des = rotateToFace(theta, r)
    theta_des = theta + wrapToPi(atan2(r(2),r(1)) - theta);
end

== matlab function MPC/PhaseSpace Filter Code/Subsystem3/MATLAB Function ==
  data: dt input; z input; x output; P output; u input; x input; P input; V input; mRED parameter; IRED parameter; V output
function [x, P,V] = fcn(dt, z, u, x, P, V, mRED, IRED)
Q = blkdiag(0.0001*eye(2), 0.0000001);
R = 0.0000001*eye(3);
rho = 0.995;
Fargs.m = mRED;
Fargs.I = IRED;

% --- PREDICT ---------------------------------------------------------
[xk, F, G] = dyn(x,  dt, u, Fargs);
Pk         = F*P*F' + G*Q*G';

% --- For no Measurments ----------------------------------------------
if ~isfinite(z)
    x = xk;
    P = Pk;
    return
end

% --- Measurement -----------------------------------------------------
[zPred, H] = meas(xk, []);
y          = z - zPred;

% --- Angle Innovation (wrapped difference) ---------------------------
y(3) =  attErr(z(3),zPred(3));

% --- Strong Tracking -------------------------------------------------
% if det(V) == 0
%     V = rho*y*y';
% else
%     V = rho*(rho*V + y*y') / (1 + rho);
% end
% 
% L = corrP4Q(Pk, H, R, V);
% Pk = L*Pk*L';

% --- UPDATE ----------------------------------------------------------
S          = H*Pk*H' + R;
K          = Pk* H' / S;

corr       = K*y;
x          = xk + corr;
I          = eye(size(K,1));
P          = (I - K*H)*Pk*(I - K*H)' + K*R*K';

end

function [x,F,G] = dyn(x, dt, u, Fargs)
    F = [eye(3), dt*eye(3);
         zeros(3), eye(3)];

    m = diag([1/Fargs.m; 1/Fargs.m; 1/Fargs.I]);

    G = [(dt^2/2)*m; dt*m];

    x = F*x + G*u;
end

function [z, H] = meas(x, hargs)
    % H = eye(6);
    H = [eye(3), zeros(3)];
    z = H*x;
end

function e_out = attErr(ref,act)
Ax = [cos(act) sin(act); -sin(act) cos(act)]*[1;0];
Rx = [cos(ref) sin(ref); -sin(ref) cos(ref)]*[1;0];
Ry = [cos(ref) sin(ref); -sin(ref) cos(ref)]*[0;1];

e_in = Rx - Ax;

a = sign(Ry'*e_in);
e_out = -a*norm(e_in);
end

function L = corrP4Q(P_k, H, R, V)
    % Inputs:
    % P_K    - Time Updated Covar
    % H      - Measurement Jacobian
    % R      - Measurement covar
    % V      - True Pzz
    %
    % Find lambda Matrix
    % Initial guess for Lambda
    n = length(P_k);
    Lambda0 = ones(n/2,1); % Starting with an identity scaled by 2

    % Solve using Levenberg-Marquardt
    options = optimoptions('lsqnonlin', 'Algorithm', 'levenberg-marquardt','display','off');
    lb = ones(n/2,1);
    % Call lsqnonlin.
    Lambda_sol = lsqnonlin(@(x) objFun(x, eye(3), P_k, H, R, V), Lambda0, lb, [], options);
    L = blkdiag(diag(Lambda_sol(1:3)), ...
                     diag(Lambda_sol(1:3)));
end

function res = objFun(diagLambda, Izz, P, H, R, V)
    % Convert the vector of diagonal entries into a diagonal matrix Lambda.
    Lambda = blkdiag(diag(diagLambda(1:3)), ...
                     diag(diagLambda(1:3)));
    
    % Update the state covariance using the matrix fading factor.
    P_new = Lambda * P * Lambda;
    
    % Compute the measurement covariance.
    Pzz = H * P_new * H' + R;
    
    % Compute the residual. The goal is to have Pzz^{-1} * V as close as possible
    % to the identity Izz.
    % (Depending on your filter design, you may have a different function to minimize.)
    resMat = Izz - inv(Pzz) * V;
    
    % Return the residual as a vector (by stacking the matrix columns).
    res = resMat(:);
end

== matlab function MPC/2 - Guidance/Default APF PPL (BLACK)/MATLAB Function ==
  data: desiredPosition input; currentPosition output; currentPosition input; obstacles input; attractiveGain input; repulsiveGain input; influenceRange input; angularGain input; baseRate parameter
function currentPosition = APFPathPlanner(desiredPosition, currentPosition, obstacles, attractiveGain, repulsiveGain, influenceRange, angularGain, baseRate)
    % APFPathPlanner for real-time path planning in Simulink
    % Controls X, Y, and Attitude (Theta)
    % currentPosition: [x, y, theta]
    % desiredPosition: [x, y, theta]
    % obstacles: Nx2 matrix of obstacle positions [x, y]
    % attractiveGain: Scalar for attractive force
    % repulsiveGain: Scalar for repulsive force
    % influenceRange: Scalar, range for obstacle influence
    % angularGain: Scalar for angular adjustment


    % Position control for X and Y
    attractiveForce = attractiveGain * (desiredPosition(1:2) - currentPosition(1:2));
    repulsiveForce = zeros(1, 2);

    % % Repulsive force from obstacles
    for i = 1:size(obstacles, 1)
        obstaclePos = obstacles(i, :);
        distanceToObstacle = norm(currentPosition(1:2) - obstaclePos);

        if distanceToObstacle < influenceRange
            directionFromObstacle = (currentPosition(1:2) - obstaclePos) / distanceToObstacle;
            magnitude = repulsiveGain * (1 / distanceToObstacle - 1 / influenceRange) * (1 / distanceToObstacle^2);
            repulsiveForce = repulsiveForce + magnitude * directionFromObstacle;
        end
    end

    % Combine attractive and repulsive forces
    totalForce = attractiveForce + repulsiveForce;

    % Update X and Y position
    deltaT = baseRate;
    newPosition = currentPosition(1:2) + deltaT * totalForce;

    % Attitude control for Theta
    angularDifference = atan2(sin(desiredPosition(3) - currentPosition(3)), cos(desiredPosition(3) - currentPosition(3)));
    newTheta = currentPosition(3) + angularGain * angularDifference * deltaT;

    % Normalize newTheta to be within -pi to pi
    newTheta = atan2(sin(newTheta), cos(newTheta));

    % Update currentPosition with new position and attitude
    currentPosition = [newPosition, newTheta];

end

== matlab function MPC/PhaseSpace Filter Code/Subsystem1/MATLAB Function ==
  data: dt input; z input; x output; P output; u input; x input; P input; V input; mBLACK parameter; IBLACK parameter; V output
function [x, P,V] = fcn(dt, z, u, x, P, V, mBLACK, IBLACK)
Q = blkdiag(0.0001*eye(2), 0.0000001);
R = 0.0000001*eye(3);
rho = 0.995;
Fargs.m = mBLACK;
Fargs.I = IBLACK;

% --- PREDICT ---------------------------------------------------------
[xk, F, G] = dyn(x,  dt, u, Fargs);
Pk         = F*P*F' + G*Q*G';

% --- For no Measurments ----------------------------------------------
if ~isfinite(z)
    x = xk;
    P = Pk;
    return
end

% --- Measurement -----------------------------------------------------
[zPred, H] = meas(xk, []);
y          = z - zPred;

% --- Angle Innovation (wrapped difference) ---------------------------
y(3) =  attErr(z(3),zPred(3));

% --- Strong Tracking -------------------------------------------------
% if det(V) == 0
%     V = rho*y*y';
% else
%     V = rho*(rho*V + y*y') / (1 + rho);
% end
% 
% L = corrP4Q(Pk, H, R, V);
% Pk = L*Pk*L';

% --- UPDATE ----------------------------------------------------------
S          = H*Pk*H' + R;
K          = Pk* H' / S;

corr       = K*y;
x          = xk + corr;
I          = eye(size(K,1));
P          = (I - K*H)*Pk*(I - K*H)' + K*R*K';

end

function [x,F,G] = dyn(x, dt, u, Fargs)
    F = [eye(3), dt*eye(3);
         zeros(3), eye(3)];

    m = diag([1/Fargs.m; 1/Fargs.m; 1/Fargs.I]);

    G = [(dt^2/2)*m; dt*m];

    x = F*x + G*u;
end

function [z, H] = meas(x, hargs)
    % H = eye(6);
    H = [eye(3), zeros(3)];
    z = H*x;
end

function e_out = attErr(ref,act)
Ax = [cos(act) sin(act); -sin(act) cos(act)]*[1;0];
Rx = [cos(ref) sin(ref); -sin(ref) cos(ref)]*[1;0];
Ry = [cos(ref) sin(ref); -sin(ref) cos(ref)]*[0;1];

e_in = Rx - Ax;

a = sign(Ry'*e_in);
e_out = -a*norm(e_in);
end

function L = corrP4Q(P_k, H, R, V)
    % Inputs:
    % P_K    - Time Updated Covar
    % H      - Measurement Jacobian
    % R      - Measurement covar
    % V      - True Pzz
    %
    % Find lambda Matrix
    % Initial guess for Lambda
    n = length(P_k);
    Lambda0 = ones(n/2,1); % Starting with an identity scaled by 2

    % Solve using Levenberg-Marquardt
    options = optimoptions('lsqnonlin', 'Algorithm', 'levenberg-marquardt','display','off');
    lb = ones(n/2,1);
    % Call lsqnonlin.
    Lambda_sol = lsqnonlin(@(x) objFun(x, eye(3), P_k, H, R, V), Lambda0, lb, [], options);
    L = blkdiag(diag(Lambda_sol(1:3)), ...
                     diag(Lambda_sol(1:3)));
end

function res = objFun(diagLambda, Izz, P, H, R, V)
    % Convert the vector of diagonal entries into a diagonal matrix Lambda.
    Lambda = blkdiag(diag(diagLambda(1:3)), ...
                     diag(diagLambda(1:3)));
    
    % Update the state covariance using the matrix fading factor.
    P_new = Lambda * P * Lambda;
    
    % Compute the measurement covariance.
    Pzz = H * P_new * H' + R;
    
    % Compute the residual. The goal is to have Pzz^{-1} * V as close as possible
    % to the identity Izz.
    % (Depending on your filter design, you may have a different function to minimize.)
    resMat = Izz - inv(Pzz) * V;
    
    % Return the residual as a vector (by stacking the matrix columns).
    res = resMat(:);
end
